simulink model "L0405"  (Simulink 10.2)
settings: Solver=ode45  StartTime=0.0  StopTime=30  MaxStep=0.01  RelTol=1e-3
libraries: simulink x5
settings Model: LogicAnalyzerSignalOrdering=35e2f5c9-5eff-4630-a3cf-9e8b07e8781d  Creator=Ranci  LastModifiedBy=Ranci
settings DataIOCC: SaveFormat=Dataset  SignalLoggingSaveFormat=Dataset  ReturnWorkspaceOutputs=on
settings OptimizationCC: LifeSpan=auto
settings DebuggingCC: UnderspecifiedInitializationDetection=Simplified  MergeDetectMultiDrivingBlocksExec=error  FcnCallInpInsideContextMsg=error  SFUnexpectedBacktrackingDiag=error  SFNoUnconditionalDefaultTransitionDiag=error  SFExecutionAtInitializationDiag=warning  ArithmeticOperatorsInVariantConditions=error
settings HardwareCC: ProdBitPerPointer=64  ProdBitPerSizeT=64  ProdBitPerPtrDiffT=64  ProdLargestAtomicFloat=Float  ProdIntDivRoundTo=Zero  ProdEndianess=LittleEndian  ProdWordSize=64  ProdHWDeviceType=Intel->x86-64 (Windows64)
settings ModelReferenceCC: PropagateSignalLabelsOutOfModel=on
settings SFSimCC: SimUseLocalCustomCode=on  CustomCodeUndefinedFunction=FilterOut
settings RTWCC: RTWUseLocalCustomCode=on
settings CodeAppCC: StateflowObjectComments=off
settings GRTTargetCC: TargetLangStandard=C99 (ISO)  CombineOutputUpdateFcns=on  GRTInterface=off
settings ConfigComp: CovMetricSettings=dwe  CovSaveCumulativeToWorkspaceVar=off  CovSaveSingleToWorkspaceVar=off  CovExternalEMLEnable=on

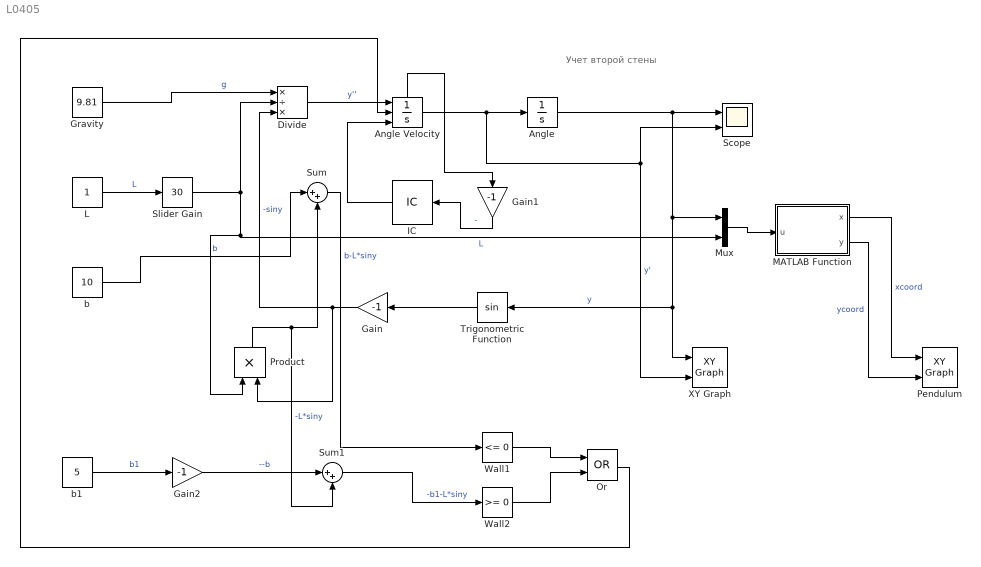
== system L0405 ==
  note: Учет второй стены
  Angle : Integrator
  Angle Velocity : Integrator  ExternalReset=rising  InitialConditionSource=external  InitialCondition=2  ShowStatePort=on
  Divide : Product  Inputs=*/*
  Gain : Gain  Gain=-1
  Gain1 : Gain  Gain=-1
  Gain2 : Gain  Gain=-1
  Gravity : Constant  Value=9.81
  IC : InitialCondition  Value=2
  L : Constant
  MATLAB Function : MATLAB Function  TreatAsAtomicUnit=on
  Mux : Mux  Inputs=2
  Or : Logic  Operator=OR  AllPortsSameDT=off  OutDataTypeStr=boolean
  Pendulum : simulink/Sinks/XY Graph  xmin=-30  xmax=30  ymin=-30  ymax=30  st=-1
  Product : Product
  Scope : Scope  NumInputPorts=2
  Slider Gain : simulink/Math Operations/Slider Gain  gain=30  low=0  high=30
  Sum : Sum  Inputs=|++
  Sum1 : Sum  Inputs=|++
  Trigonometric Function : Trigonometry
  Wall1 : simulink/Logic and Bit Operations/Compare To Zero  relop=<=  OutDataTypeStr=boolean
  Wall2 : simulink/Logic and Bit Operations/Compare To Zero  relop=>=  OutDataTypeStr=boolean
  XY Graph : simulink/Sinks/XY Graph  xmin=-4  xmax=4  ymin=-2  ymax=2  st=-1
  b : Constant  Value=10
  b1 : Constant  Value=5
  wires:
  L/1 -> Slider Gain/1  "L"
  Gravity/1 -> Divide/1  "g"
  Slider Gain/1 -> Divide/2, Product/1, Mux/2  "L"
  Divide/1 -> Angle Velocity/1  "y''"
  Angle Velocity/1 -> XY Graph/2, Scope/2, Angle/1  "y'"
  Angle/1 -> Mux/1, XY Graph/1, Trigonometric Function/1, Scope/1  "y"
  Trigonometric Function/1 -> Gain/1
  Gain/1 -> Product/2, Divide/3  "-siny"
  Mux/1 -> MATLAB Function/1(u)
  MATLAB Function/1(x) -> Pendulum/1  "xcoord"
  MATLAB Function/2(y) -> Pendulum/2  "ycoord"
  b/1 -> Sum/1  "b"
  Product/1 -> Sum1/2, Sum/2  "-L*siny"
  Angle Velocity/State -> Gain1/1
  Gain1/1 -> IC/1  "-"
  IC/1 -> Angle Velocity/3
  Gain2/1 -> Sum1/1  "--b"
  Sum1/1 -> Wall2/1  "-b1-L*siny"
  Sum/1 -> Wall1/1  "b-L*siny"
  Wall1/1 -> Or/1
  Wall2/1 -> Or/2
  Or/1 -> Angle Velocity/2
  b1/1 -> Gain2/1  "b1"

== matlab function MATLAB Function ==
  data: x output double; u input double; y output double
function [x, y] = fcn(u)
x = u(2) * sin(u(1));      %координата х
y = -u(2) * cos(u(1));     %координата y
